simulink model "verify_Vapour_Pressure_mdl"  (R2016b)
settings: Solver=VariableStepDiscrete  StartTime=0.0  StopTime=10  MaxStep=0.1  RelTol=1e-3  EnableMultiTasking=on
libraries: carnot x2, simulink x1
settings Model: Creator=drhf  LastModifiedBy=srrt
settings DataIOCC: LimitDataPoints=on  SaveFormat=Array
settings OptimizationCC: ExpressionDepthLimit=2147483647  LifeSpan=inf
settings DebuggingCC: UnderspecifiedInitializationDetection=Classic  MergeDetectMultiDrivingBlocksExec=none  SolverPrmCheckMsg=warning  StateNameClashWarn=warning  SFUnexpectedBacktrackingDiag=warning  SFNoUnconditionalDefaultTransitionDiag=warning  SFExecutionAtInitializationDiag=none
settings HardwareCC: ProdBitPerPointer=32  ProdBitPerSizeT=32  ProdBitPerPtrDiffT=32  ProdLargestAtomicFloat=None  ProdIntDivRoundTo=Undefined  ProdEndianess=Unspecified  ProdWordSize=32  ProdHWDeviceType=32-bit Generic
settings ModelReferenceCC: PropagateSignalLabelsOutOfModel=off
settings GRTTargetCC: TargetLangStandard=C89/C90 (ANSI)  GeneratePreprocessorConditionals=Disable all  CombineOutputUpdateFcns=off  GRTInterface=on
settings ConfigComp: CovMetricSettings=dw  CovHtmlReporting=on  CovSaveCumulativeToWorkspaceVar=on  CovSaveSingleToWorkspaceVar=on  CovExternalEMLEnable=off

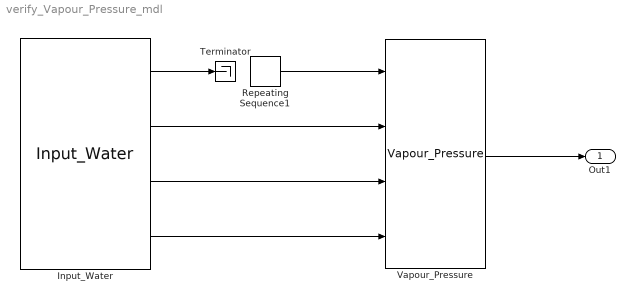
== system verify_Vapour_Pressure_mdl ==
  Input_Water : carnot/Basic/Material_Properties/Input_Water  T=20  p=1e5  xd=0
  Repeating Sequence1 : simulink/Sources/Repeating Sequence  rep_seq_t=[0:10 11]  rep_seq_y=[0.01 5:5:50 50]
  Terminator : Terminator
  Vapour_Pressure : carnot/Basic/Material_Properties/Vapour_Pressure  VariantControl=CarlibClassic  INPUTARGUMENTS=state variables (classic)  DEBUGLEVEL=WARNINGLEVEL  MAXTOTALMESSAGES=inf  MAXCONSECUTIVEMESSAGES=inf  WRITETOFILE=0  FILENAME='errors.txt'
  Out1 : Outport
  wires:
  Vapour_Pressure/1 -> Out1/1
  Repeating Sequence1/1 -> Vapour_Pressure/1
  Input_Water/1 -> Terminator/1
  Input_Water/3 -> Vapour_Pressure/3
  Input_Water/2 -> Vapour_Pressure/2
  Input_Water/4 -> Vapour_Pressure/4
